simulink model "confstate_policy_test"  (R2019a)
settings: Solver=FixedStepAuto  StartTime=0.0  StopTime=10  FixedStep=1e-3  RelTol=1e-3
settings Model: Creator=trangvu  LastModifiedBy=marceca

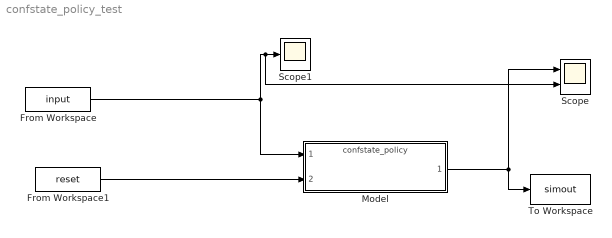
== system confstate_policy_test ==
  From Workspace : FromWorkspace  VariableName=input  SampleTime=0
  From Workspace1 : FromWorkspace  VariableName=reset  SampleTime=0
  Model : ModelReference  ModelNameDialog=confstate_policy.slx  SimulationMode=Normal  ModelReferenceVersion=1.749  SimulationMode=Normal
  Scope : Scope  NumInputPorts=2
  Scope1 : Scope
  To Workspace : ToWorkspace  VariableName=simout  SaveFormat=Timeseries  SampleTime=-1
  wires:
  From Workspace/1 -> Scope/2, Scope1/1, Model/1
  Model/1 -> To Workspace/1, Scope/1
  From Workspace1/1 -> Model/2
